simulink model "Model_no_simx"  (R2020b)
settings: Solver=VariableStepAuto  StartTime=0.0  StopTime=10  FixedStep=0.1  RelTol=1e-3
model workspace (MAT data in the model file):
  l1 = Simulink.Parameter
  l1.Value = 0.3
  l1.Description = '"Bicep length"'
  l1.DataType = 'auto'
  l1.Dimensions = [1 1]
  l2 = Simulink.Parameter
  l2.Value = 0.3
  l2.Description = '"Forearm length"'
  l2.DataType = 'auto'
  l2.Dimensions = [1 1]
libraries: simulink_extras x1, pid_lib x1
settings Model: PacingRate=0.500000  OrderedModelArguments=off  Creator=Luke Bidulka  LastModifiedBy=ndroz

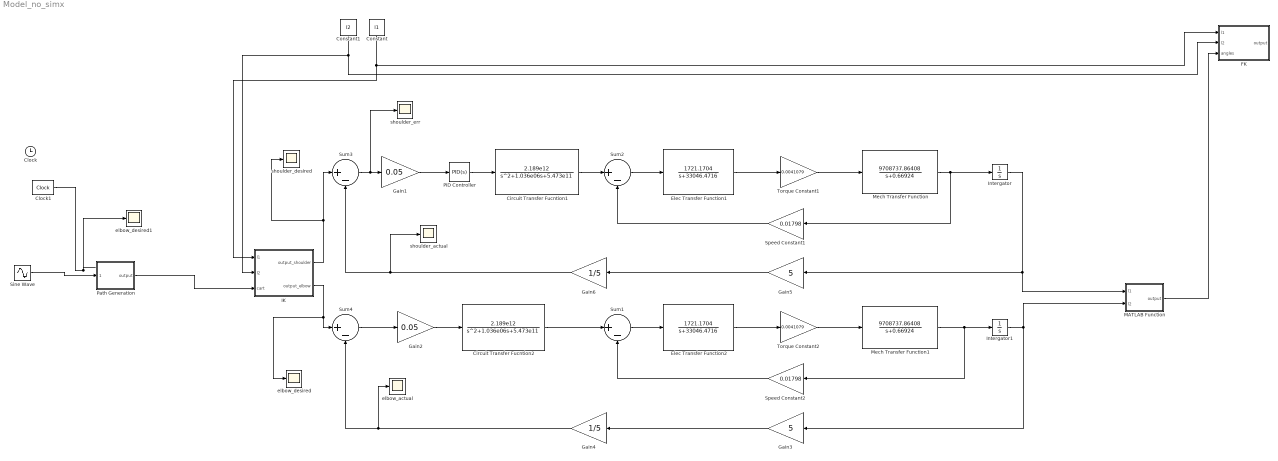
== system Model_no_simx ==
  Circuit Transfer Fucntion1 : TransferFcn  Numerator=[2.189e12]  Denominator=[1 1.036e06 5.473e11]
  Circuit Transfer Fucntion2 : TransferFcn  Numerator=[2.189e12]  Denominator=[1 1.036e06 5.473e11]
  Clock : Clock
  Clock1 : simulink_extras/Flip Flops/Clock  period=0.01
  Constant : Constant  Value=l1
  Constant1 : Constant  Value=l2
  Elec Transfer Function1 : TransferFcn  Numerator=[1721.1704]  Denominator=[1 33046.4716]
  Elec Transfer Function2 : TransferFcn  Numerator=[1721.1704]  Denominator=[1 33046.4716]
  FK : MATLAB Function  TreatAsAtomicUnit=on
  Gain1 : Gain  Gain=0.05
  Gain2 : Gain  Gain=0.05
  Gain3 : Gain  Gain=5
  Gain4 : Gain  Gain=1/5
  Gain5 : Gain  Gain=5
  Gain6 : Gain  Gain=1/5
  IK : MATLAB Function  TreatAsAtomicUnit=on
  Intergator : Integrator
  Intergator1 : Integrator
  MATLAB Function : MATLAB Function  TreatAsAtomicUnit=on
  Mech Transfer Function : TransferFcn  Numerator=[9708737.86408]  Denominator=[1 0.66924]
  Mech Transfer Function1 : TransferFcn  Numerator=[9708737.86408]  Denominator=[1 0.66924]
  PID Controller : pid_lib/PID Controller  Controller=PID  Form=Parallel  TimeDomain=Continuous-time  UseExternalTs=off  SampleTime=-1  IntegratorMethod=Forward Euler  FilterMethod=Forward Euler  ControllerParametersSource=internal  P=1  I=1  D=0  UseFilter=on  N=100  TunerSelectOption=Transfer Function Based (PID Tuner App)  InitialConditionSource=internal  InitialConditionForIntegrator=0  InitialConditionForFilter=0  DifferentiatorICPrevScaledInput=0  ExternalReset=none  TrackingMode=off  Kt=1  LimitOutput=off  SatLimitsSource=internal  UpperSaturationLimit=inf  LowerSaturationLimit=-inf  LinearizeAsGain=on  AntiWindupMode=none  Kb=1  POutMin=[]  POutMax=[]  IOutMin=[]  IOutMax=[]  DOutMin=[]  DOutMax=[]  NOutMin=[]  NOutMax=[]  SumOutMin=[]  SumOutMax=[]  SaturationOutMin=[]  SaturationOutMax=[]  PParamMin=[]  PParamMax=[]  IParamMin=[]  IParamMax=[]  DParamMin=[]  DParamMax=[]  NParamMin=[]  NParamMax=[]  KbParamMin=[]  KbParamMax=[]  KtParamMin=[]  KtParamMax=[]  KbOutMin=[]  KbOutMax=[]  KtOutMin=[]  KtOutMax=[]  IntegratorOutMin=[]  IntegratorOutMax=[]  FilterOutMin=[]  FilterOutMax=[]  SumI1OutMin=[]  SumI1OutMax=[]  SumI2OutMin=[]  SumI2OutMax=[]  SumI3OutMin=[]  SumI3OutMax=[]  SumI4OutMin=[]  SumI4OutMax=[]  SumDOutMin=[]  SumDOutMax=[]  DifferentiatorOutMin=[]  DifferentiatorOutMax=[]  FilterDiffOutCoefMin=[]  FilterDiffOutCoefMax=[]  ReciprocalOutMin=[]  ReciprocalOutMax=[]  SumDenOutMin=[]  SumDenOutMax=[]  SumNumOutMin=[]  SumNumOutMax=[]  DivideOutMin=[]  DivideOutMax=[]  UdiffTsProdOutMin=[]  UdiffTsProdOutMax=[]  NTsProdOutMin=[]  NTsProdOutMax=[]  UintegralTsProdOutMin=[]  UintegralTsProdOutMax=[]  UngainTsProdOutMin=[]  UngainTsProdOutMax=[]  IntegratorContinuousStateAttributes=''  IntegratorStateMustResolveToSignalObject=off  IntegratorRTWStateStorageClass=Auto  FilterContinuousStateAttributes=''  FilterStateMustResolveToSignalObject=off  FilterRTWStateStorageClass=Auto  ParallelPVariant=InternalParameters  IdealPVariant=Disabled  IVariant=InternalParameters  DVariant=InternalParameters  IntegratorVariant=Continuous  SatVariant=Disabled  AWVariant=Passthrough  PCopyVariant=Disabled  TRVariant=Disabled  FdbkBlocksVariant=Forward  IdealPFdbkVariant=Disabled  SatFdbkVariant=Disabled  DerivativeFilterVariant=ContFilter  NVariant=InternalParameters  NCopyVariant=Disabled  FilterICVariant=InternalICsFilter  IntegratorICVariant=InternalICs  ExternalResetVariant=Disabled  TRSumVariant=Passthrough  SumFdbkVariant=Disabled  SumVariant=Sum_PID  TsampFilterVariant=InternalTs  TsampNgainVariant=Passthrough  TsampIntegralVariant=Passthrough  ExternalSaturationOutDataTypeStr=Inherit: Same as second input
  Path Generation : MATLAB Function  TreatAsAtomicUnit=on
  Sine Wave : Sin  SampleTime=0.05
  Speed Constant1 : Gain  Gain=0.01798
  Speed Constant2 : Gain  Gain=0.01798
  Sum{1..4} (4 alike) : Sum  Inputs=|+-
  Torque Constant1 : Gain  Gain=0.0041079
  Torque Constant2 : Gain  Gain=0.0041079
  elbow_actual : Scope
  elbow_desired : Scope
  elbow_desired1 : Scope
  shoulder_actual : Scope
  shoulder_desired : Scope
  shoulder_err : Scope
  wires:
  Path Generation/1(output) -> IK/3(cart)
  Constant1/1 -> FK/2(l2), IK/2(l2)
  Constant/1 -> FK/1(l1), IK/1(l1)
  Gain5/1 -> Gain6/1
  Elec Transfer Function1/1 -> Torque Constant1/1
  Circuit Transfer Fucntion1/1 -> Sum2/1
  Speed Constant1/1 -> Sum2/2
  Sum2/1 -> Elec Transfer Function1/1
  Sum3/1 -> shoulder_err/1, Gain1/1
  Gain2/1 -> Circuit Transfer Fucntion2/1
  Elec Transfer Function2/1 -> Torque Constant2/1
  Speed Constant2/1 -> Sum1/2
  Gain3/1 -> Gain4/1
  Sum4/1 -> Gain2/1
  Sum1/1 -> Elec Transfer Function2/1
  Circuit Transfer Fucntion2/1 -> Sum1/1
  Gain4/1 -> elbow_actual/1, Sum4/2
  IK/1(output_shoulder) -> shoulder_desired/1, Sum3/1
  IK/2(output_elbow) -> elbow_desired/1, Sum4/1
  MATLAB Function/1(output) -> FK/3(angles)
  Gain6/1 -> shoulder_actual/1, Sum3/2
  Gain1/1 -> PID Controller/1
  PID Controller/1 -> Circuit Transfer Fucntion1/1
  Torque Constant1/1 -> Mech Transfer Function/1
  Mech Transfer Function/1 -> Intergator/1, Speed Constant1/1
  Intergator/1 -> MATLAB Function/1(l1), Gain5/1
  Torque Constant2/1 -> Mech Transfer Function1/1
  Mech Transfer Function1/1 -> Speed Constant2/1, Intergator1/1
  Intergator1/1 -> Gain3/1, MATLAB Function/2(l2)
  Clock1/1 -> elbow_desired1/1
  Sine Wave/1 -> Path Generation/1(sampleTime)

== matlab function Model_no_simx/FK ==
  data: l1 input; l2 input; angles input; output output
% Fwd Kinematics
function output = Fwd_Kin(l1, l2, angles)

    q0 = angles(1); % Configuration-space shoulder angle
    q1 = angles(2); % Configuration-space elbow angle

    % Get task-space coordinates
    x = l1*cos(q0) + l2*cos(q0+q1);
    y = l1*sin(q0) + l2*sin(q0+q1);

    % Output the task-space cartesian coordinats
    output = [x;y];

end

== matlab function Model_no_simx/IK ==
  data: l1 input; l2 input; cart input; output_shoulder output; output_elbow output
% Inv Kinematics
function [output_shoulder,output_elbow] = Inv_Kin(l1, l2, cart)
    x = cart(1); % Task-space x coord
    y = cart(2); % Task-space y coord

    % Get q1 first, need it to calculate q0. We will always
    % take the "right-handed" solution where q1 is (+). 
    q1 = abs(acos((x^2 + y^2 - l1^2 - l2^2)/(2*l1*l2)));

    % Get q0
    gamma = atan(y/x);
    beta = atan((l2*sin(q1))/(l1 + l2*cos(q1)));

    q0 = gamma - beta;
    
    % Ouput our angle vector
    output_shoulder = q0;
    output_elbow = q1;
    
end

== matlab function Model_no_simx/Path Generation ==
  settings: updateMethod=DISCRETE  sampleTime=0.2
  data: output output; sampleTime input
function output = path_gen(sampleTime)

    % Define the trajectory, a circle (r = 0.15) over 10sec
    t = (0:0.1:10)'; % Time
    %count = length(t);
    center = [0.3 0.1];
    radius = 0.15;
    theta = t*(2*pi/t(end));
    
    circ_path_points = zeros(length(t),2);
    
    persistent count more_count;
   
    
    if isempty(count)
        count = double(1);
        more_count = 1;
    end
    
    more_count = more_count + 1;

    for i = 1:length(theta)
        circ_path_points(i,:) = center + radius*[cos(theta(i)) sin(theta(i))];
    end   
    
    path_points = [0.2 0.4; 0.2 0.4; 0.2 0.4; 0.2 0.4; 0.2 0.4; 0.2 0.4];
    
    %output = circ_path_points(count,:);
    output = path_points(count,:);
end

== matlab function Model_no_simx/MATLAB Function ==
  data: l1 input; output output; l2 input
function output = Combine(l1, l2)
    % Ouput our angle vector
    output = [l1; l2];
    
end
